simulink model "gm_detect_rising_edge"  (R2017a)
settings: Solver=FixedStepAuto  StartTime=0.0  StopTime=10.0  RelTol=1e-3
libraries: simulink x1
settings Model: Creator=mini  LastModifiedBy=mini
settings OptimizationCC: BlockReduction=off  ConditionallyExecuteInputs=off
settings DebuggingCC: InheritedTsInSrcMsg=none  SingleTaskRateTransMsg=error

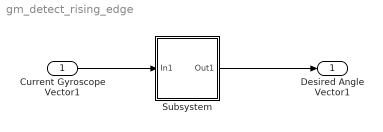
== system gm_detect_rising_edge ==
  Current Gyroscope Vector1 : Inport  OutDataTypeStr=boolean
  Subsystem : Subsystem
  Desired Angle Vector1 : Outport  OutDataTypeStr=boolean
  wires:
  Subsystem/1(Out1) -> Desired Angle Vector1/1
  Current Gyroscope Vector1/1 -> Subsystem/1(In1)

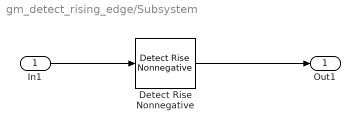
== system gm_detect_rising_edge/Subsystem ==
  In1 : Inport  OutDataTypeStr=boolean
  Detect Rise Nonnegative : simulink/Logic and Bit Operations/Detect Rise Nonnegative  vinit=0  OutDataTypeStr=boolean
      settings: SourceProductName=Simulink  SourceProductBaseCode=SL
  Out1 : Outport  OutDataTypeStr=boolean
  wires:
  In1/1 -> Detect Rise Nonnegative/1
  Detect Rise Nonnegative/1 -> Out1/1
